simulink subsystem "Driver"  (R2024b)
settings: Solver=VariableStepAuto  StartTime=0.0  StopTime=10.0  RelTol=1e-3
settings Model: Creator=Ian  LastModifiedBy=Ian

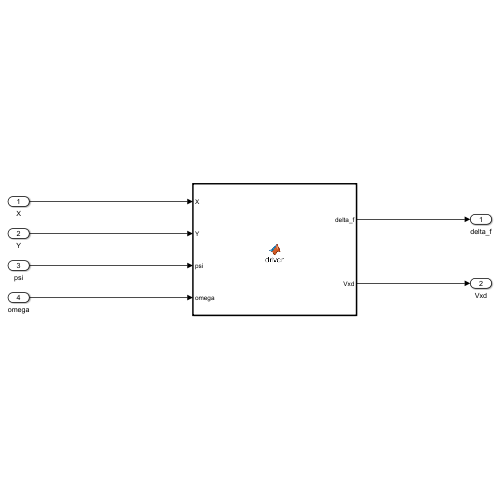
[thumbnail: Simulink's stored preview of the top-level diagram]
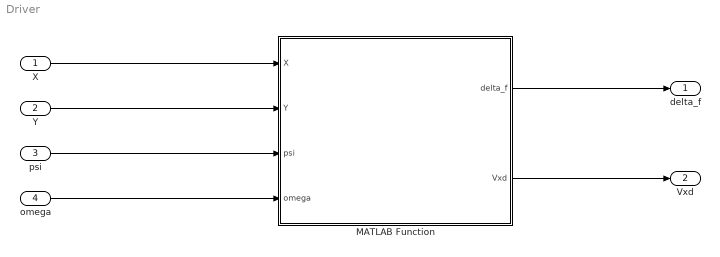
== system Driver ==
  X : Inport
  Y : Inport  Port=2
  psi : Inport  Port=3
  omega : Inport  Port=4
  MATLAB Function : MATLAB Function  TreatAsAtomicUnit=on
  delta_f : Outport
  Vxd : Outport  Port=2
  wires:
  Y/1 -> MATLAB Function/2(Y)
  MATLAB Function/1(delta_f) -> delta_f/1
  X/1 -> MATLAB Function/1(X)
  MATLAB Function/2(Vxd) -> Vxd/1
  psi/1 -> MATLAB Function/3(psi)
  omega/1 -> MATLAB Function/4(omega)

== matlab function Driver/MATLAB Function ==
  data: X input; delta_f output; Y input; psi input; omega input; Vxd output
function [delta_f, Vxd] = driver(X, Y, psi, omega)
    
    % Load track data (x_ref, y_ref, psi_ref)
    persistent track_x track_y track_psi;
    if isempty(track_x)
        run('Project2Week2Code.m');
    end

    L = 2.5; 
    Kp = 0.5;  % gain for lateral error; utilizing controller 
    Kd = 0.3;  % gain for heading error
    Kw = 0.1;  % gain for yaw rate damping
    Vmax = 5; % Max speed

    % Find nearest track point
    [~, idx] = min((track_x - X).^2 + (track_y - Y).^2);
    X_ref = track_x(idx);
    Y_ref = track_y(idx);
    psi_ref = track_psi(idx);

    ey = Y - Y_ref;
    epsi = psi - psi_ref;

    delta_f = -Kp * ey - Kd * epsi - Kw * omega;
    
    Vxd = Vmax * (1 - 0.5 * abs(epsi));

    % Bound constraints
    delta_f = max(min(delta_f, 0.5), -0.5);
    Vxd = max(Vxd, 2); 
end
